simulink model "testing_SVM"  (Simulink 7.9)
settings: Solver=ode45  StartTime=0.0  StopTime=1  RelTol=1e-3
libraries: simulink x6
settings Model: Creator=Dmitriy  LastModifiedBy=Dmitriy

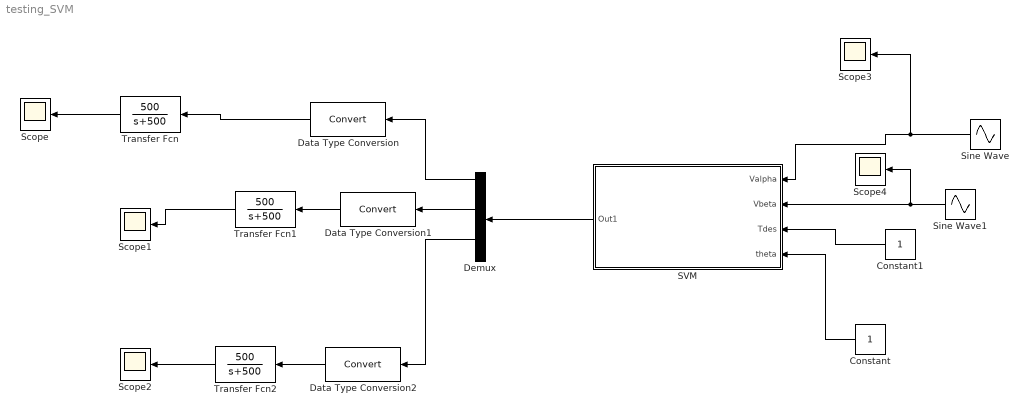
== system testing_SVM ==
  Constant : Constant
  Constant1 : Constant
  Data Type Conversion : DataTypeConversion
  Data Type Conversion1 : DataTypeConversion
  Data Type Conversion2 : DataTypeConversion
  Demux : Demux  Outputs=6
  SVM : Subsystem  SystemSampleTime=10^-6
  Scope{,1..4} (5 alike) : Scope
      Scope2 settings: SaveName=ScopeData2
      Scope3 settings: SaveName=ScopeData4
      Scope4 settings: SaveName=ScopeData5
  Sine Wave : Sin  Amplitude=10  Frequency=20  SampleTime=0
  Sine Wave1 : Sin  Amplitude=10  Frequency=20  Phase=pi/2  SampleTime=0
  Transfer Fcn : TransferFcn  Numerator=[500]  Denominator=[1 500]
  Transfer Fcn1 : TransferFcn  Numerator=[500]  Denominator=[1 500]
  Transfer Fcn2 : TransferFcn  Numerator=[500]  Denominator=[1 500]
  wires:
  SVM/1(Out1) -> Demux/1
  Sine Wave/1 -> SVM/1(Valpha), Scope3/1
  Sine Wave1/1 -> SVM/2(Vbeta), Scope4/1
  Constant/1 -> SVM/4(theta)
  Constant1/1 -> SVM/3(Tdes)
  Demux/1 -> Data Type Conversion/1
  Demux/3 -> Data Type Conversion1/1
  Demux/5 -> Data Type Conversion2/1
  Data Type Conversion/1 -> Transfer Fcn/1
  Transfer Fcn/1 -> Scope/1
  Transfer Fcn1/1 -> Scope1/1
  Data Type Conversion1/1 -> Transfer Fcn1/1
  Data Type Conversion2/1 -> Transfer Fcn2/1
  Transfer Fcn2/1 -> Scope2/1

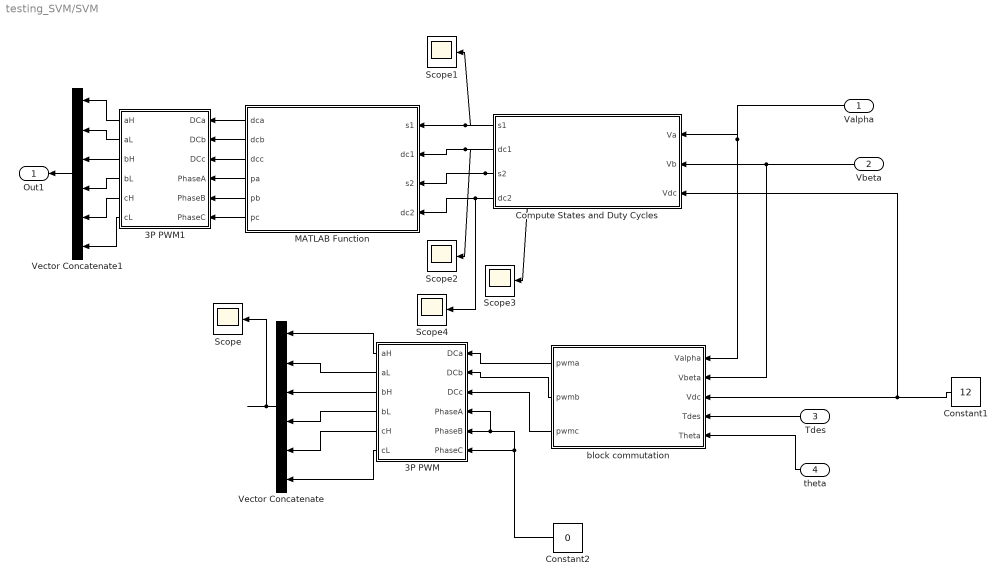
== system testing_SVM/SVM ==
  Valpha : Inport
  Vbeta : Inport  Port=2
  Tdes : Inport  Port=3
  theta : Inport  Port=4
  3P PWM : Subsystem  TreatAsAtomicUnit=on  SystemSampleTime=1
  3P PWM1 : Subsystem  TreatAsAtomicUnit=on  SystemSampleTime=10^-6
  Compute States and Duty Cycles : MATLAB Function  TreatAsAtomicUnit=on  SystemSampleTime=.001
  Constant1 : Constant  Value=12
  Constant2 : Constant  Value=0
  MATLAB Function : MATLAB Function  TreatAsAtomicUnit=on  SystemSampleTime=10^-6
  Scope{,1..4} (5 alike) : Scope
      Scope settings: SaveName=ScopeData3
      Scope1 settings: SaveName=ScopeData6
      Scope2 settings: SaveName=ScopeData7
      Scope3 settings: SaveName=ScopeData8
      Scope4 settings: SaveName=ScopeData9
  Vector Concatenate : Concatenate  NumInputs=6
  Vector Concatenate1 : Concatenate  NumInputs=6
  block commutation : MATLAB Function  TreatAsAtomicUnit=on  SystemSampleTime=1
  Out1 : Outport
  wires:
  Valpha/1 -> block commutation/1(Valpha), Compute States and Duty Cycles/1(Va)
  Vbeta/1 -> block commutation/2(Vbeta), Compute States and Duty Cycles/2(Vb)
  Constant1/1 -> block commutation/3(Vdc), Compute States and Duty Cycles/3(Vdc)
  Tdes/1 -> block commutation/4(Tdes)
  theta/1 -> block commutation/5(Theta)
  block commutation/2(pwmb) -> 3P PWM/2(DCb)
  block commutation/3(pwmc) -> 3P PWM/3(DCc)
  block commutation/1(pwma) -> 3P PWM/1(DCa)
  3P PWM/1(aH) -> Vector Concatenate/1
  3P PWM/2(aL) -> Vector Concatenate/2
  3P PWM/3(bH) -> Vector Concatenate/3
  3P PWM/4(bL) -> Vector Concatenate/4
  3P PWM/5(cH) -> Vector Concatenate/5
  3P PWM/6(cL) -> Vector Concatenate/6
  Vector Concatenate/1 -> Scope/1
  Constant2/1 -> 3P PWM/6(PhaseC), 3P PWM/5(PhaseB), 3P PWM/4(PhaseA)
  MATLAB Function/1(dca) -> 3P PWM1/1(DCa)
  MATLAB Function/2(dcb) -> 3P PWM1/2(DCb)
  MATLAB Function/3(dcc) -> 3P PWM1/3(DCc)
  MATLAB Function/4(pa) -> 3P PWM1/4(PhaseA)
  MATLAB Function/5(pb) -> 3P PWM1/5(PhaseB)
  MATLAB Function/6(pc) -> 3P PWM1/6(PhaseC)
  3P PWM1/1(aH) -> Vector Concatenate1/1
  3P PWM1/2(aL) -> Vector Concatenate1/2
  3P PWM1/3(bH) -> Vector Concatenate1/3
  3P PWM1/4(bL) -> Vector Concatenate1/4
  3P PWM1/5(cH) -> Vector Concatenate1/5
  3P PWM1/6(cL) -> Vector Concatenate1/6
  Compute States and Duty Cycles/1(s1) -> MATLAB Function/1(s1), Scope1/1
  Compute States and Duty Cycles/2(dc1) -> MATLAB Function/2(dc1), Scope2/1
  Compute States and Duty Cycles/3(s2) -> MATLAB Function/3(s2), Scope3/1
  Compute States and Duty Cycles/4(dc2) -> MATLAB Function/4(dc2), Scope4/1
  Vector Concatenate1/1 -> Out1/1

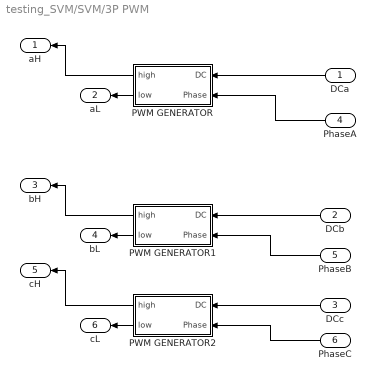
== system testing_SVM/SVM/3P PWM ==
  DCa : Inport
  DCb : Inport  Port=2
  DCc : Inport  Port=3
  PhaseA : Inport  Port=4
  PhaseB : Inport  Port=5
  PhaseC : Inport  Port=6
  PWM GENERATOR : Subsystem  TreatAsAtomicUnit=on
      settings: ErrorFcn=10^6
  PWM GENERATOR1 : Subsystem  TreatAsAtomicUnit=on
  PWM GENERATOR2 : Subsystem  TreatAsAtomicUnit=on
  aH : Outport
  aL : Outport  Port=2
  bH : Outport  Port=3
  bL : Outport  Port=4
  cH : Outport  Port=5
  cL : Outport  Port=6
  wires:
  DCa/1 -> PWM GENERATOR/1(DC)
  PWM GENERATOR/1(high) -> aH/1
  PWM GENERATOR/2(low) -> aL/1
  DCb/1 -> PWM GENERATOR1/1(DC)
  PWM GENERATOR1/1(high) -> bH/1
  PWM GENERATOR1/2(low) -> bL/1
  DCc/1 -> PWM GENERATOR2/1(DC)
  PWM GENERATOR2/1(high) -> cH/1
  PWM GENERATOR2/2(low) -> cL/1
  PhaseA/1 -> PWM GENERATOR/2(Phase)
  PhaseB/1 -> PWM GENERATOR1/2(Phase)
  PhaseC/1 -> PWM GENERATOR2/2(Phase)

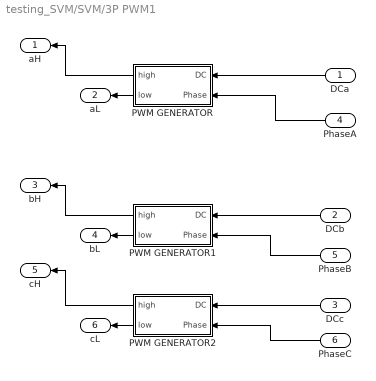
== system testing_SVM/SVM/3P PWM1 ==
  DCa : Inport
  DCb : Inport  Port=2
  DCc : Inport  Port=3
  PhaseA : Inport  Port=4
  PhaseB : Inport  Port=5
  PhaseC : Inport  Port=6
  PWM GENERATOR : Subsystem  TreatAsAtomicUnit=on
      settings: ErrorFcn=10^6
  PWM GENERATOR1 : Subsystem  TreatAsAtomicUnit=on
  PWM GENERATOR2 : Subsystem  TreatAsAtomicUnit=on
  aH : Outport
  aL : Outport  Port=2
  bH : Outport  Port=3
  bL : Outport  Port=4
  cH : Outport  Port=5
  cL : Outport  Port=6
  wires:
  DCa/1 -> PWM GENERATOR/1(DC)
  PWM GENERATOR/1(high) -> aH/1
  PWM GENERATOR/2(low) -> aL/1
  DCb/1 -> PWM GENERATOR1/1(DC)
  PWM GENERATOR1/1(high) -> bH/1
  PWM GENERATOR1/2(low) -> bL/1
  DCc/1 -> PWM GENERATOR2/1(DC)
  PWM GENERATOR2/1(high) -> cH/1
  PWM GENERATOR2/2(low) -> cL/1
  PhaseA/1 -> PWM GENERATOR/2(Phase)
  PhaseB/1 -> PWM GENERATOR1/2(Phase)
  PhaseC/1 -> PWM GENERATOR2/2(Phase)

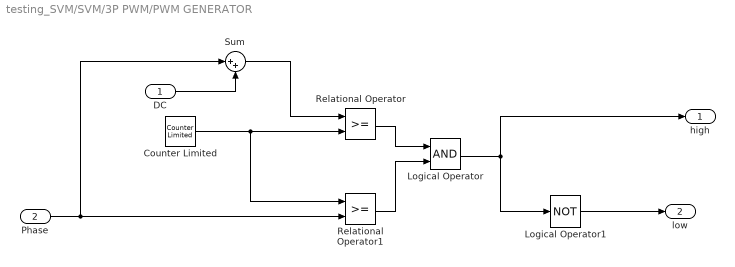
== system testing_SVM/SVM/3P PWM/PWM GENERATOR ==
  DC : Inport
  Phase : Inport  Port=2
  Counter Limited : simulink/Sources/Counter Limited  uplimit=1000  tsamp=-1
  Logical Operator : Logic  AllPortsSameDT=off  OutDataTypeStr=boolean
  Logical Operator1 : Logic  Operator=NOT  AllPortsSameDT=off  OutDataTypeStr=boolean
  Relational Operator : RelationalOperator  OutDataTypeStr=boolean
  Relational Operator1 : RelationalOperator  OutDataTypeStr=boolean
  Sum : Sum  Inputs=|++
  high : Outport
  low : Outport  Port=2
  wires:
  Counter Limited/1 -> Relational Operator/2, Relational Operator1/1
  Phase/1 -> Relational Operator1/2, Sum/1
  DC/1 -> Sum/2
  Sum/1 -> Relational Operator/1
  Relational Operator/1 -> Logical Operator/1
  Relational Operator1/1 -> Logical Operator/2
  Logical Operator/1 -> Logical Operator1/1, high/1
  Logical Operator1/1 -> low/1

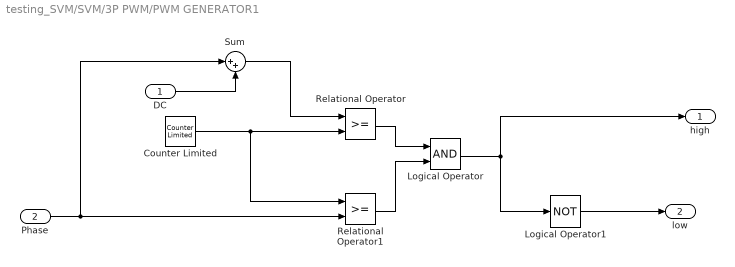
== system testing_SVM/SVM/3P PWM/PWM GENERATOR1 ==
  DC : Inport
  Phase : Inport  Port=2
  Counter Limited : simulink/Sources/Counter Limited  uplimit=1000  tsamp=-1
  Logical Operator : Logic  AllPortsSameDT=off  OutDataTypeStr=boolean
  Logical Operator1 : Logic  Operator=NOT  AllPortsSameDT=off  OutDataTypeStr=boolean
  Relational Operator : RelationalOperator  OutDataTypeStr=boolean
  Relational Operator1 : RelationalOperator  OutDataTypeStr=boolean
  Sum : Sum  Inputs=|++
  high : Outport
  low : Outport  Port=2
  wires:
  Counter Limited/1 -> Relational Operator/2, Relational Operator1/1
  Phase/1 -> Relational Operator1/2, Sum/1
  DC/1 -> Sum/2
  Sum/1 -> Relational Operator/1
  Relational Operator/1 -> Logical Operator/1
  Relational Operator1/1 -> Logical Operator/2
  Logical Operator/1 -> Logical Operator1/1, high/1
  Logical Operator1/1 -> low/1

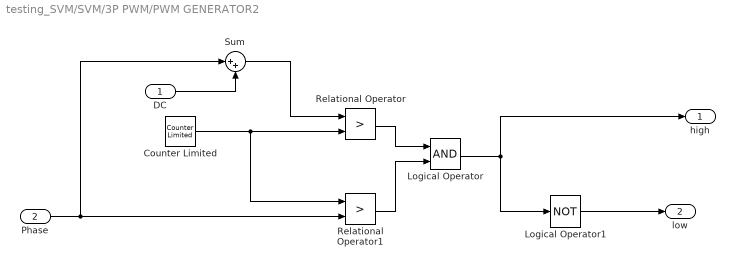
== system testing_SVM/SVM/3P PWM/PWM GENERATOR2 ==
  DC : Inport
  Phase : Inport  Port=2
  Counter Limited : simulink/Sources/Counter Limited  uplimit=1000  tsamp=-1
  Logical Operator : Logic  AllPortsSameDT=off  OutDataTypeStr=boolean
  Logical Operator1 : Logic  Operator=NOT  AllPortsSameDT=off  OutDataTypeStr=boolean
  Relational Operator : RelationalOperator  Operator=>  OutDataTypeStr=boolean
  Relational Operator1 : RelationalOperator  Operator=>  OutDataTypeStr=boolean
  Sum : Sum  Inputs=|++
  high : Outport
  low : Outport  Port=2
  wires:
  Counter Limited/1 -> Relational Operator/2, Relational Operator1/1
  Phase/1 -> Relational Operator1/2, Sum/1
  DC/1 -> Sum/2
  Sum/1 -> Relational Operator/1
  Relational Operator/1 -> Logical Operator/1
  Relational Operator1/1 -> Logical Operator/2
  Logical Operator/1 -> Logical Operator1/1, high/1
  Logical Operator1/1 -> low/1

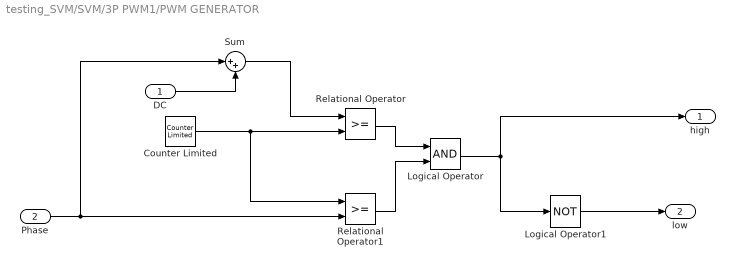
== system testing_SVM/SVM/3P PWM1/PWM GENERATOR ==
  DC : Inport
  Phase : Inport  Port=2
  Counter Limited : simulink/Sources/Counter Limited  uplimit=1000  tsamp=-1
  Logical Operator : Logic  AllPortsSameDT=off  OutDataTypeStr=boolean
  Logical Operator1 : Logic  Operator=NOT  AllPortsSameDT=off  OutDataTypeStr=boolean
  Relational Operator : RelationalOperator  OutDataTypeStr=boolean
  Relational Operator1 : RelationalOperator  OutDataTypeStr=boolean
  Sum : Sum  Inputs=|++
  high : Outport
  low : Outport  Port=2
  wires:
  Counter Limited/1 -> Relational Operator/2, Relational Operator1/1
  Phase/1 -> Relational Operator1/2, Sum/1
  DC/1 -> Sum/2
  Sum/1 -> Relational Operator/1
  Relational Operator/1 -> Logical Operator/1
  Relational Operator1/1 -> Logical Operator/2
  Logical Operator/1 -> Logical Operator1/1, high/1
  Logical Operator1/1 -> low/1

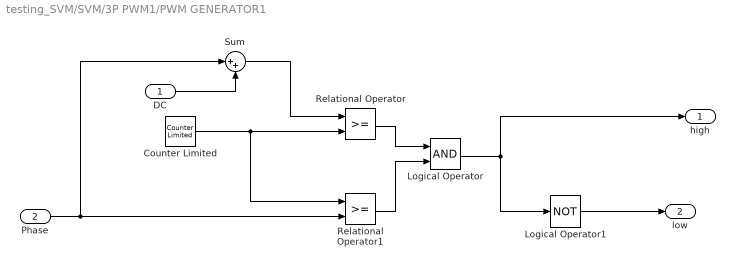
== system testing_SVM/SVM/3P PWM1/PWM GENERATOR1 ==
  DC : Inport
  Phase : Inport  Port=2
  Counter Limited : simulink/Sources/Counter Limited  uplimit=1000  tsamp=-1
  Logical Operator : Logic  AllPortsSameDT=off  OutDataTypeStr=boolean
  Logical Operator1 : Logic  Operator=NOT  AllPortsSameDT=off  OutDataTypeStr=boolean
  Relational Operator : RelationalOperator  OutDataTypeStr=boolean
  Relational Operator1 : RelationalOperator  OutDataTypeStr=boolean
  Sum : Sum  Inputs=|++
  high : Outport
  low : Outport  Port=2
  wires:
  Counter Limited/1 -> Relational Operator/2, Relational Operator1/1
  Phase/1 -> Relational Operator1/2, Sum/1
  DC/1 -> Sum/2
  Sum/1 -> Relational Operator/1
  Relational Operator/1 -> Logical Operator/1
  Relational Operator1/1 -> Logical Operator/2
  Logical Operator/1 -> Logical Operator1/1, high/1
  Logical Operator1/1 -> low/1

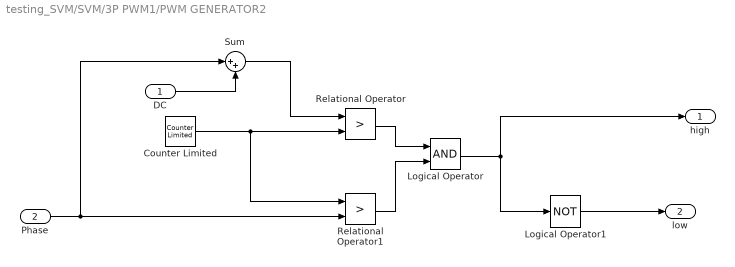
== system testing_SVM/SVM/3P PWM1/PWM GENERATOR2 ==
  DC : Inport
  Phase : Inport  Port=2
  Counter Limited : simulink/Sources/Counter Limited  uplimit=1000  tsamp=-1
  Logical Operator : Logic  AllPortsSameDT=off  OutDataTypeStr=boolean
  Logical Operator1 : Logic  Operator=NOT  AllPortsSameDT=off  OutDataTypeStr=boolean
  Relational Operator : RelationalOperator  Operator=>  OutDataTypeStr=boolean
  Relational Operator1 : RelationalOperator  Operator=>  OutDataTypeStr=boolean
  Sum : Sum  Inputs=|++
  high : Outport
  low : Outport  Port=2
  wires:
  Counter Limited/1 -> Relational Operator/2, Relational Operator1/1
  Phase/1 -> Relational Operator1/2, Sum/1
  DC/1 -> Sum/2
  Sum/1 -> Relational Operator/1
  Relational Operator/1 -> Logical Operator/1
  Relational Operator1/1 -> Logical Operator/2
  Logical Operator/1 -> Logical Operator1/1, high/1
  Logical Operator1/1 -> low/1

== matlab function SVM/block commutation ==
  data: Valpha input double; pwma output double; Vbeta input double; Vdc input double; Tdes input double; Theta input double; pwmb output double; pwmc output double
function [pwma,pwmb,pwmc]  = block_com(Valpha,Vbeta,Vdc,Tdes,Theta)
%#codegen

ang = floor(Theta/(pi/3));

d = sqrt(Valpha^2+Vbeta^2)/Vdc;
d = 1;


switch ang
    case 0
        if(Tdes>=0)
            %s2
            pwms = [d d 0];
        else
            %s1
            pwms = [d 0 0];
        end
    case 1
        if(Tdes>=0)
            %s3
            pwms = [0 d 0];
        else
            %s2
            pwms = [d d 0];
        end
        
    case 2
        if(Tdes>=0)
            %s4
            pwms = [0 d d];
        else
            %s3
            pwms = [0 d 0];
        end
    case 3
        if(Tdes>=0)
            %s5
            pwms = [0 0 d];
        else
            %s4
            pwms = [0 d d];
        end
    case 4
        if(Tdes>=0)
            %s6
            pwms = [d 0 d];
        else
            %s5
            pwms = [0 0 d];
        end
    case 5
        if(Tdes>=0)
            %s1
            pwms = [d 0 0];
        else
            %s6
            pwms = [d 0 d];
        end
        
    otherwise
        pwms = [0 0 0];
end
pwms=pwms*1000;
pwma=pwms(1);
pwmb= pwms(2);
pwmc = pwms(3);

== matlab function SVM/Compute States and Duty Cycles ==
  data: Va input double; s1 output double; dc1 output double; Vb input double; s2 output double; Vdc input double; dc2 output double
function [s1,dc1, s2, dc2] = statesAndCycles(Va,Vb, Vdc)
%#codegen
    %Given desired Valpha and Vbeta, and the supply voltage, compute the inverter states to toggle
    %between and the duty cycle of each
    
    %right now we're saying that the length of each state vector is Vdc, which
    %is probably wrong
    
    ang = wrapTo2Pi(angle(Va+1i*Vb));
    
    sext = floor(ang/(pi/3))
    
    v1 = 1 +1i;
    v2 = 1 + 1i;
    
    %states as defined in james mevey's thesis
    %v1, v2 are complex values of the voltages
    switch sext
        case 0
            s1 = 1;
            v1 = Vdc;
            
            s2 = 2;
            [t1 t2] = pol2cart(pi/3,Vdc);
            v2 = t1+1i*t2;
            
        case 1
            s1 = 2;
            [t1 t2] = pol2cart(pi/3,Vdc);
            v1 = t1+1i*t2;
            
            s2 = 3;
            [t1 t2] = pol2cart(2*pi/3,Vdc);
            v2 = t1+1i*t2;
            
        case 2
            s1 = 3;
            [t1 t2] = pol2cart(2*pi/3,Vdc);
            v1 = t1+1i*t2;
            
            s2 = 4;
            [t1 t2] = pol2cart(pi,Vdc);
            v2 = t1+1i*t2;
        case 3
            s1 = 4;
            [t1 t2] = pol2cart(pi,Vdc);
            v1 = t1+1i*t2;
            
            s2 = 5;
            [t1 t2] = pol2cart(4*pi/3,Vdc);
            v2 = t1+1i*t2;
        case 4
            s1 = 5;
            [t1 t2] = pol2cart(4*pi/3,Vdc);
            v1 = t1+1i*t2;
            
            
            s2 = 6;
            [t1 t2] = pol2cart(5*pi/3,Vdc);
            v2 = t1+1i*t2;
        case 5
            s1 = 6;
            [t1 t2] = pol2cart(5*pi/3,Vdc);
            v1 = t1+1i*t2;
            
            s2 = 1;
            v2 = Vdc;
        otherwise
            s1 = 0;
            s2 = 0;
    end
    
v1 
v2
num = Vb - imag(v1)*Va/real(v1)
den = imag(v2)-imag(v1)*real(v2)/real(v1)
dc2 = num/den;
dc1 = (Va - real(v2)*dc2)/real(v1);


    %solve for intersection of v1 line and v2 line translated to the desired
    %place
    
% 
%     num = Va-imag(v2)*Vb/real(v2)- imag(v1);
%     den = real(v1) - imag(v2)/real(v2);
%     
%     xint = num/den;
%     yint = (imag(v1)/real(v1))*xint;
%     
%     %duty cycle 1 equals length of sv1 divided by Vdc, which is nominal length
%     dc1 = sqrt(xint^2+yint^2)/Vdc;
%     
%     %duty cycle 2 is distance from the tip of sv1 to the desired point, divided
%     %by Vdc
%     
%     dc2 = sqrt((xint-Va)^2 +(yint - Vb)^2)/Vdc;

end

function lambda = wrapTo2Pi(lambda)
%wrapTo2Pi Wrap angle in radians to [0 2*pi]
%
%   lambdaWrapped = wrapTo2Pi(LAMBDA) wraps angles in LAMBDA, in radians,
%   to the interval [0 2*pi] such that zero maps to zero and 2*pi maps
%   to 2*pi. (In general, positive multiples of 2*pi map to 2*pi and
%   negative multiples of 2*pi map to zero.)
%
%   See also wrapToPi, wrapTo180, wrapTo360.

% Copyright 2007-2008 The MathWorks, Inc.
% $Revision: 1.1.6.1 $  $Date: 2008/12/22 23:50:53 $

positiveInput = (lambda > 0);
lambda = mod(lambda, 2*pi);
lambda((lambda == 0) & positiveInput) = 2*pi;
end

function p = angle(h)
%ANGLE  Phase angle.
%   ANGLE(H) returns the phase angles, in radians, of a matrix with
%   complex elements.
%
%   Class support for input X:
%      float: double, single
%
%   See also ABS, UNWRAP.

%   Copyright 1984-2010 The MathWorks, Inc.
%   $Revision: 5.7.4.2 $  $Date: 2010/04/21 21:31:19 $

p = atan2(imag(h), real(h));
end

== matlab function SVM/MATLAB Function ==
  data: s1 input double; dca output double; dc1 input double; s2 input double; dc2 input double; dcb output double; dcc output double; pa output double; pb output double; pc output double
function [dca,dcb,dcc,pa,pb,pc] = PWM_module_inputs(s1,dc1,s2,dc2)
%#codegen
%given the two states to switch between and the duty cycle of each, compute
%the proper duty cycles and phases for each leg of the half bridge. Duty
%cycles should be between 1 and 1000, as should phases. If duty cycle is
%1000, and phase is 400, then the duty cycle really only ends up being 400,
%get it? If not, look at the pwm block.

%pattern is: all low, then s1, then s2

d1 = dc1*1000;
d2 = dc2*1000;
p2 = 1000-d2;
d0 = 1000 - d1 -d2;
p0 = 0;
p1 = d0;

dca = 1000;
dcb = 1000;
dcc = 1000;

switch(s1)
    
    case 1
        pa = d0;
        if(s2==2)
            pb = d0+d1;
            pc = 1000;
        else
            pb = 1000;
            pc = d0+d1;
        end
    case 2
        pc = 1000;
        if(s2==3)
            dca = d1;
            pa = d0;
            pb = d0;
        else
            pa = d0;
            dcb = d1;
            pb = d0;
        end
    case 3
        pb = d0;
        if(s2==4)
            pa = 1000;
            pc = d0+d1;
        else
            pa = d0+d1;
            pc =1000;
        end
    case 4
        pa = 1000;
        if(s2 == 5)
            dcb = d1;
            pb = d0;
            pc = d0;
        else
            pb = d0;
            dcc = d1;
            pc = d0;
        end
    case 5
        pc = d0;
        if(s2==6)
            pa = d0+d1;
            pb = 1000;
        else
            pa = 1000;
            pb = d0+d1;
        end
    case 6
        pb=1000;
        if(s2==1)
            pa = d0;
            dcc = d1;
            pc = d0;
        else
            dca = d1;
            pa = d0;
            pc = d0;
        end
    otherwise
        pa=1000;
        pb = 1000;
        pc = 1000;
end

end
